simulink model "Sim_PA_DDPG"  (R2025a)
settings: Solver=ode1  StartTime=0.0  StopTime=Tf  FixedStep=Ts_Sim  RelTol=1e-3
values from neighbouring files (symbols this model uses):
  control_noise = 0.05    [DDPG_simulation.mat]    (also in Test_Pos_Att_DDPG.m)
  p_IC = IC(10)    [Test_Pos_Att_DDPG.m]
  phi_IC = IC(7)    [Test_Pos_Att_DDPG.m]
  psi_IC = IC(9)    [Test_Pos_Att_DDPG.m]
  q_IC = IC(11)    [Test_Pos_Att_DDPG.m]
  r_IC = IC(12)    [Test_Pos_Att_DDPG.m]
  state_noise = 0.05    [DDPG_simulation.mat]    (also in Test_Pos_Att_DDPG.m)
  theta_IC = IC(8)    [Test_Pos_Att_DDPG.m]
  Ts_Sim = 0.01    [DDPG_simulation.mat]    (also in Test_Pos_Att_DDPG.m)
  u_IC = IC(4)    [Test_Pos_Att_DDPG.m]
  v_IC = IC(5)    [Test_Pos_Att_DDPG.m]
  w_IC = IC(6)    [Test_Pos_Att_DDPG.m]
  x_IC = IC(1)    [Test_Pos_Att_DDPG.m]
  y_IC = IC(2)    [Test_Pos_Att_DDPG.m]
  z_IC = IC(3)    [Test_Pos_Att_DDPG.m]
undefined symbols (not defined in the file or in its folder): phi_limit, pqr_Limit, psi_dsr, psi_limit, saturation_logic, theta_limit, uvw_Limit, wind_logic, xy_Limit, z_Limit
libraries: rllib x2
settings Model: Creator=nt488543  LastModifiedBy=re606359

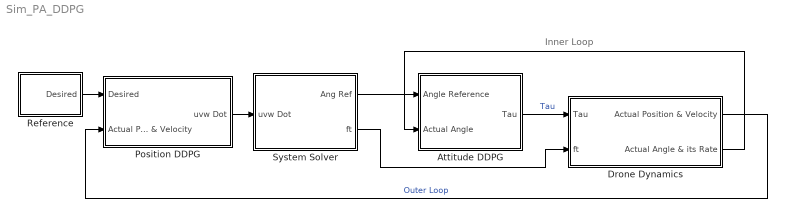
== system Sim_PA_DDPG ==
  note: Inner Loop
  Attitude DDPG : Subsystem
  Drone Dynamics : Subsystem
  Position DDPG : Subsystem
  Reference : Subsystem
  System Solver : Subsystem
  wires:
  Reference/1(Desired) -> Position DDPG/1(Desired)
  Attitude DDPG/1(Tau) -> Drone Dynamics/1(Tau)  "Tau"
  Drone Dynamics/1(Actual Position & Velocity) -> Position DDPG/2(Actual Position & Velocity)  "Outer Loop"
  Drone Dynamics/2(Actual Angle & its Rate) -> Attitude DDPG/2(Actual Angle)
  Position DDPG/1(uvw Dot) -> System Solver/1(uvw Dot)
  System Solver/1(Ang Ref) -> Attitude DDPG/1(Angle Reference)
  System Solver/2(ft) -> Drone Dynamics/2(ft)

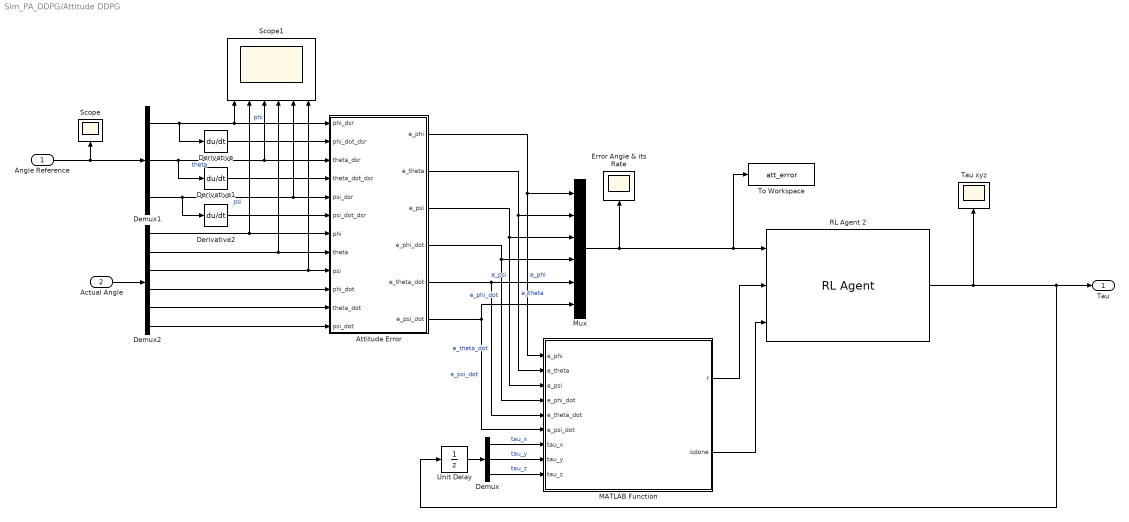
== system Sim_PA_DDPG/Attitude DDPG ==
  Angle Reference : Inport
  Actual Angle : Inport  Port=2
  Attitude Error : MATLAB Function  TreatAsAtomicUnit=on
  Demux : Demux  Outputs=3
  Demux1 : Demux  Outputs=3
  Demux2 : Demux  Outputs=6
  Derivative : Derivative
  Derivative1 : Derivative
  Derivative2 : Derivative
  Error Angle & its Rate : Scope
      settings: ActiveDisplayYMinimum=-3.5181599273654109  ActiveDisplayYMaximum=2.1435969273697308  DataLoggingVariableName=ScopeData12
  MATLAB Function : MATLAB Function  TreatAsAtomicUnit=on
  Mux : Mux  Inputs=6
  RL Agent 2 : rllib/RL Agent  Agent=agent2  ExternalActionAsInput=off  ProvideLastAction=off  ProvideCumRwd=off  TreatAsDirectFeedthrough=on  UseStrictObservationDataTypes=off
  Scope : Scope
      settings: ActiveDisplayYMinimum=-0.07573  ActiveDisplayYMaximum=0.06612  DataLoggingVariableName=ScopeData5
  Scope1 : Scope  NumInputPorts=6
      settings: ActiveDisplayYMinimum=-0.08548920227975057  ActiveDisplayYMaximum=0.079586119310867051  DataLoggingVariableName=ScopeData6
  Tau xyz : Scope
      settings: ActiveDisplayYMinimum=-2.4987406879663467  ActiveDisplayYMaximum=2.4991613775491714  DataLoggingVariableName=ScopeData11
  To Workspace : ToWorkspace  VariableName=att_error  SampleTime=Ts_Sim
  Unit Delay : UnitDelay  SampleTime=Ts_Sim  HasFrameUpgradeWarning=on
  Tau : Outport
  wires:
  MATLAB Function/1(r) -> RL Agent 2/2
  Mux/1 -> To Workspace/1, RL Agent 2/1, Error Angle & its Rate/1
  Attitude Error/1(e_phi) -> Mux/1, MATLAB Function/1(e_phi)  "e_phi"
  Attitude Error/2(e_theta) -> Mux/2, MATLAB Function/2(e_theta)  "e_theta"
  Attitude Error/3(e_psi) -> Mux/3, MATLAB Function/3(e_psi)  "e_psi"
  Attitude Error/4(e_phi_dot) -> Mux/4, MATLAB Function/4(e_phi_dot)  "e_phi_dot"
  Attitude Error/5(e_theta_dot) -> MATLAB Function/5(e_theta_dot), Mux/5  "e_theta_dot"
  Attitude Error/6(e_psi_dot) -> MATLAB Function/6(e_psi_dot), Mux/6  "e_psi_dot"
  MATLAB Function/2(isdone) -> RL Agent 2/3
  Demux/1 -> MATLAB Function/7(tau_x)  "tau_x"
  Demux/2 -> MATLAB Function/8(tau_y)  "tau_y"
  Demux/3 -> MATLAB Function/9(tau_z)  "tau_z"
  RL Agent 2/1 -> Unit Delay/1, Tau/1, Tau xyz/1
  Demux2/1 -> Scope1/2, Attitude Error/7(phi)
  Demux2/2 -> Scope1/4, Attitude Error/8(theta)
  Demux2/3 -> Attitude Error/9(psi), Scope1/6
  Demux2/4 -> Attitude Error/10(phi_dot)
  Demux2/5 -> Attitude Error/11(theta_dot)
  Demux2/6 -> Attitude Error/12(psi_dot)
  Actual Angle/1 -> Demux2/1
  Unit Delay/1 -> Demux/1
  Demux1/1 -> Derivative/1, Attitude Error/1(phi_dsr), Scope1/1  "phi"
  Demux1/3 -> Derivative2/1, Attitude Error/5(psi_dsr), Scope1/5  "psi"
  Demux1/2 -> Derivative1/1, Attitude Error/3(theta_dsr), Scope1/3  "theta"
  Angle Reference/1 -> Demux1/1, Scope/1
  Derivative/1 -> Attitude Error/2(phi_dot_dsr)
  Derivative1/1 -> Attitude Error/4(theta_dot_dsr)
  Derivative2/1 -> Attitude Error/6(psi_dot_dsr)

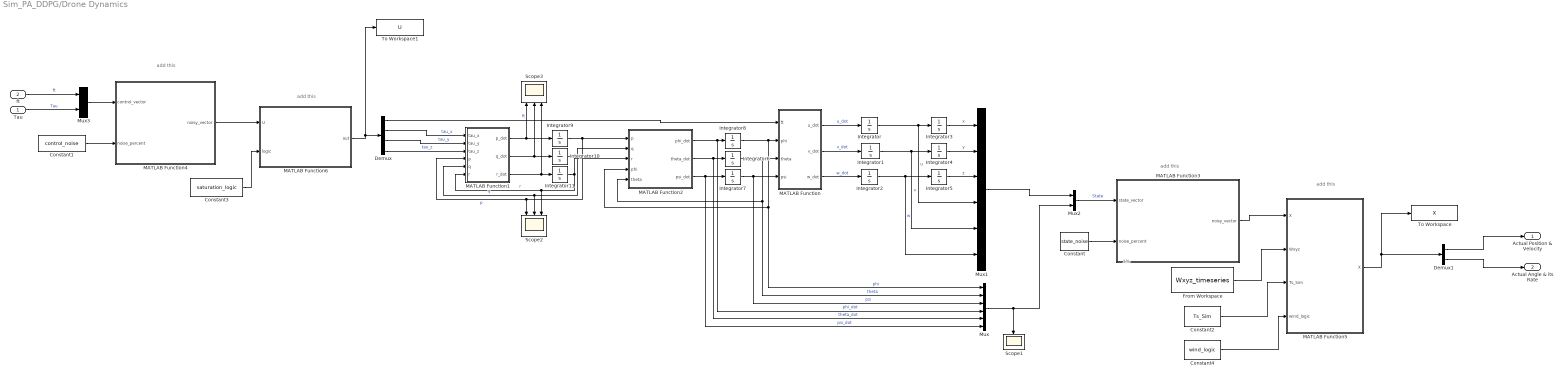
== system Sim_PA_DDPG/Drone Dynamics ==
  note: add this
  note: 1%
  note: add this
  note: add this
  note: add this
  Tau : Inport
  ft : Inport  Port=2
  Constant : Constant  Value=state_noise  SampleTime=Ts_Sim
  Constant1 : Constant  Value=control_noise
  Constant2 : Constant  Value=Ts_Sim
  Constant3 : Constant  Value=saturation_logic  SampleTime=Ts_Sim
  Constant4 : Constant  Value=wind_logic
  Demux : Demux
  Demux1 : Demux  Outputs=2
  From Workspace : FromWorkspace  VariableName=Wxyz_timeseries  SampleTime=Ts_Sim
  Integrator : Integrator  InitialCondition=u_IC  UpperSaturationLimit=uvw_Limit  LowerSaturationLimit=-uvw_Limit
  Integrator1 : Integrator  InitialCondition=v_IC  UpperSaturationLimit=uvw_Limit  LowerSaturationLimit=-uvw_Limit
  Integrator10 : Integrator  InitialCondition=q_IC  UpperSaturationLimit=pqr_Limit  LowerSaturationLimit=-pqr_Limit
  Integrator11 : Integrator  InitialCondition=r_IC  UpperSaturationLimit=pqr_Limit  LowerSaturationLimit=-pqr_Limit
  Integrator2 : Integrator  InitialCondition=w_IC  UpperSaturationLimit=uvw_Limit  LowerSaturationLimit=-uvw_Limit
  Integrator3 : Integrator  InitialCondition=x_IC  UpperSaturationLimit=xy_Limit  LowerSaturationLimit=-xy_Limit
  Integrator4 : Integrator  InitialCondition=y_IC  UpperSaturationLimit=xy_Limit  LowerSaturationLimit=-xy_Limit
  Integrator5 : Integrator  InitialCondition=z_IC  UpperSaturationLimit=z_Limit  LowerSaturationLimit=-z_Limit
  Integrator6 : Integrator  InitialCondition=theta_IC  UpperSaturationLimit=theta_limit  LowerSaturationLimit=-theta_limit  WrappedStateUpperValue=pi/2  WrappedStateLowerValue=-pi/2
  Integrator7 : Integrator  InitialCondition=psi_IC  UpperSaturationLimit=psi_limit  LowerSaturationLimit=-psi_limit
  Integrator8 : Integrator  InitialCondition=phi_IC  UpperSaturationLimit=phi_limit  LowerSaturationLimit=-phi_limit
  Integrator9 : Integrator  InitialCondition=p_IC  UpperSaturationLimit=pqr_Limit  LowerSaturationLimit=-pqr_Limit
  MATLAB Function : MATLAB Function  TreatAsAtomicUnit=on
  MATLAB Function1 : MATLAB Function  TreatAsAtomicUnit=on
  MATLAB Function2 : MATLAB Function  TreatAsAtomicUnit=on
  MATLAB Function3 : MATLAB Function  TreatAsAtomicUnit=on
  MATLAB Function4 : MATLAB Function  TreatAsAtomicUnit=on
  MATLAB Function5 : MATLAB Function  TreatAsAtomicUnit=on
  MATLAB Function6 : MATLAB Function  TreatAsAtomicUnit=on
  Mux : Mux  Inputs=6
  Mux1 : Mux  Inputs=6
  Mux2 : Mux  Inputs=2
  Mux3 : Mux  Inputs=2
  Scope1 : Scope
      settings: ActiveDisplayYMinimum=-0.79782557910284335  ActiveDisplayYMaximum=0.70695961840012789  DataLoggingVariableName=ScopeData2
  Scope2 : Scope  NumInputPorts=3
      settings: ActiveDisplayYMinimum=-0.95183  ActiveDisplayYMaximum=0.89979  DataLoggingVariableName=ScopeData3
  Scope3 : Scope  NumInputPorts=3
      settings: ActiveDisplayYMinimum=-1  ActiveDisplayYMaximum=1  DataLoggingVariableName=ScopeData4
  To Workspace : ToWorkspace  VariableName=X  SampleTime=Ts_Sim
  To Workspace1 : ToWorkspace  VariableName=U  SampleTime=Ts_Sim
  Actual Position & Velocity : Outport
  Actual Angle & its Rate : Outport  Port=2
  wires:
  Integrator4/1 -> Mux1/2  "y"
  MATLAB Function1/3(r_dot) -> Scope3/3, Integrator11/1
  MATLAB Function1/1(p_dot) -> Scope3/1, Integrator9/1
  Integrator3/1 -> Mux1/1  "x"
  Integrator5/1 -> Mux1/3  "z"
  Integrator1/1 -> Mux1/5, Integrator4/1  "v"
  ft/1 -> Mux3/1  "ft"
  Demux/3 -> MATLAB Function1/2(tau_y)  "tau_y"
  Integrator9/1 -> MATLAB Function1/4(p), Scope2/1, MATLAB Function2/1(p)  "p"
  Integrator11/1 -> MATLAB Function1/6(r), Scope2/3, MATLAB Function2/3(r)  "r"
  Integrator2/1 -> Mux1/6, Integrator5/1  "w"
  Integrator/1 -> Mux1/4, Integrator3/1  "u"
  Tau/1 -> Mux3/2  "Tau"
  Integrator7/1 -> Mux/3, MATLAB Function/4(psi)  "psi"
  Integrator8/1 -> Mux/1, MATLAB Function2/4(phi), MATLAB Function/2(phi)  "phi"
  Integrator6/1 -> MATLAB Function/3(theta), Mux/2, MATLAB Function2/5(theta)  "theta"
  Integrator10/1 -> MATLAB Function2/2(q), MATLAB Function1/5(q), Scope2/2  "q"
  Demux/4 -> MATLAB Function1/3(tau_z)  "tau_z"
  Mux/1 -> Scope1/1, Mux2/2
  MATLAB Function/3(w_dot) -> Integrator2/1  "w_dot"
  MATLAB Function/1(u_dot) -> Integrator/1  "u_dot"
  MATLAB Function/2(v_dot) -> Integrator1/1  "v_dot"
  MATLAB Function1/2(q_dot) -> Scope3/2, Integrator10/1
  Demux/2 -> MATLAB Function1/1(tau_x)  "tau_x"
  MATLAB Function2/1(phi_dot) -> Mux/4, Integrator8/1  "phi_dot"
  MATLAB Function2/2(theta_dot) -> Mux/5, Integrator6/1  "theta_dot"
  MATLAB Function2/3(psi_dot) -> Mux/6, Integrator7/1  "psi_dot"
  Mux2/1 -> MATLAB Function3/1(state_vector)  "State"
  MATLAB Function3/1(noisy_vector) -> MATLAB Function5/1("X ")
  Mux1/1 -> Mux2/1
  Constant/1 -> MATLAB Function3/2(noise_percent)
  Mux3/1 -> MATLAB Function4/1(control_vector)
  Constant1/1 -> MATLAB Function4/2(noise_percent)
  MATLAB Function4/1(noisy_vector) -> MATLAB Function6/1(U)
  Demux/1 -> MATLAB Function/1(ft)  "ft"
  From Workspace/1 -> MATLAB Function5/2(Wxyz)
  Demux1/2 -> Actual Angle & its Rate/1
  Demux1/1 -> Actual Position & Velocity/1
  Constant2/1 -> MATLAB Function5/3(Ts_Sim)
  MATLAB Function5/1(X) -> To Workspace/1, Demux1/1
  MATLAB Function6/1(out) -> To Workspace1/1, Demux/1
  Constant3/1 -> MATLAB Function6/2(logic)
  Constant4/1 -> MATLAB Function5/4(wind_logic)

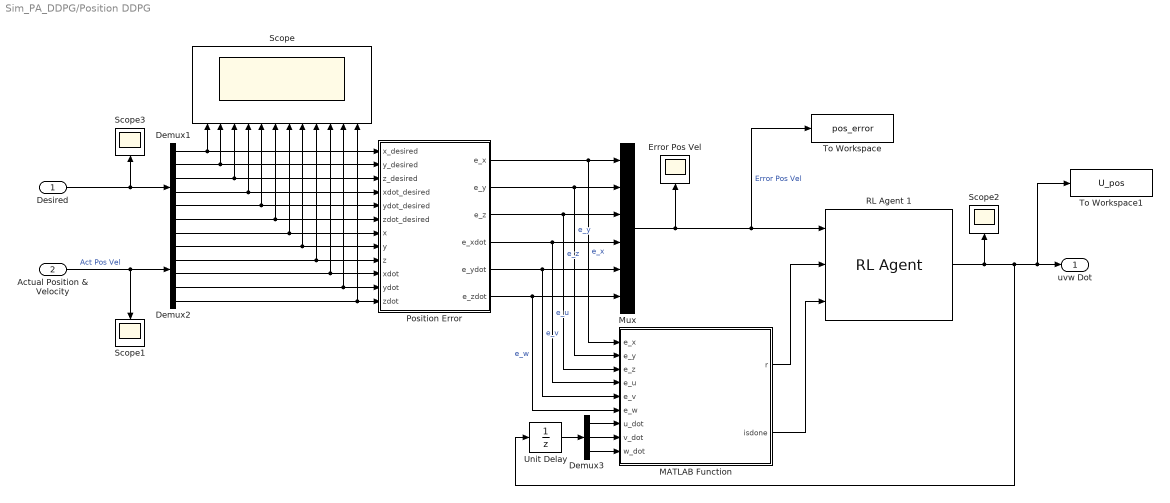
== system Sim_PA_DDPG/Position DDPG ==
  Desired : Inport
  Actual Position & Velocity : Inport  Port=2
  Demux1 : Demux  Outputs=6
  Demux2 : Demux  Outputs=6
  Demux3 : Demux  Outputs=3
  Error Pos Vel : Scope
      settings: ActiveDisplayYMinimum=-1.3710264936743408  ActiveDisplayYMaximum=0.56946492466600562  DataLoggingVariableName=Error
  MATLAB Function : MATLAB Function  TreatAsAtomicUnit=on
  Mux : Mux  Inputs=6
  Position Error : MATLAB Function  TreatAsAtomicUnit=on
  RL Agent 1 : rllib/RL Agent  Agent=agent  ExternalActionAsInput=off  ProvideLastAction=off  ProvideCumRwd=off  TreatAsDirectFeedthrough=on  UseStrictObservationDataTypes=off
  Scope : Scope  NumInputPorts=12
      settings: ActiveDisplayYMinimum=-64.8105630976365  ActiveDisplayYMaximum=12.296113517917625  DataLoggingVariableName=Difference
  Scope1 : Scope
      settings: ActiveDisplayYMinimum=-34.05865723917438  ActiveDisplayYMaximum=6.4948745222233439  DataLoggingVariableName=Actual
  Scope2 : Scope
      settings: ActiveDisplayYMinimum=-2.3417  ActiveDisplayYMaximum=1.0752  DataLoggingVariableName=ScopeData4
  Scope3 : Scope
      settings: ActiveDisplayYMinimum=-34.036737735877395  ActiveDisplayYMaximum=6.4906396228965306  DataLoggingVariableName=Ref
  To Workspace : ToWorkspace  VariableName=pos_error  SampleTime=Ts_Sim
  To Workspace1 : ToWorkspace  VariableName=U_pos  SampleTime=Ts_Sim
  Unit Delay : UnitDelay  SampleTime=Ts_Sim  HasFrameUpgradeWarning=on
  uvw Dot : Outport
  wires:
  MATLAB Function/1(r) -> RL Agent 1/2
  Mux/1 -> To Workspace/1, RL Agent 1/1, Error Pos Vel/1  "Error Pos Vel"
  RL Agent 1/1 -> To Workspace1/1, uvw Dot/1, Unit Delay/1, Scope2/1
  Position Error/1(e_x) -> MATLAB Function/1(e_x), Mux/1  "e_x"
  Position Error/2(e_y) -> MATLAB Function/2(e_y), Mux/2  "e_y"
  Position Error/3(e_z) -> Mux/3, MATLAB Function/3(e_z)  "e_z"
  Position Error/4(e_xdot) -> MATLAB Function/4(e_u), Mux/4  "e_u"
  Position Error/5(e_ydot) -> MATLAB Function/5(e_v), Mux/5  "e_v"
  Position Error/6(e_zdot) -> MATLAB Function/6(e_w), Mux/6  "e_w"
  MATLAB Function/2(isdone) -> RL Agent 1/3
  Demux1/1 -> Position Error/1(x_desired), Scope/1
  Demux1/2 -> Position Error/2(y_desired), Scope/2
  Demux1/3 -> Position Error/3(z_desired), Scope/3
  Demux1/4 -> Position Error/4(xdot_desired), Scope/4
  Demux1/5 -> Position Error/5(ydot_desired), Scope/5
  Demux1/6 -> Position Error/6(zdot_desired), Scope/6
  Desired/1 -> Scope3/1, Demux1/1
  Demux2/1 -> Position Error/7(x), Scope/7
  Demux2/2 -> Position Error/8(y), Scope/8
  Demux2/3 -> Position Error/9(z), Scope/9
  Demux2/4 -> Position Error/10(xdot), Scope/10
  Demux2/5 -> Position Error/11(ydot), Scope/11
  Demux2/6 -> Scope/12, Position Error/12(zdot)
  Actual Position & Velocity/1 -> Demux2/1, Scope1/1  "Act Pos Vel"
  Demux3/1 -> MATLAB Function/7(u_dot)
  Demux3/2 -> MATLAB Function/8(v_dot)
  Demux3/3 -> MATLAB Function/9(w_dot)
  Unit Delay/1 -> Demux3/1

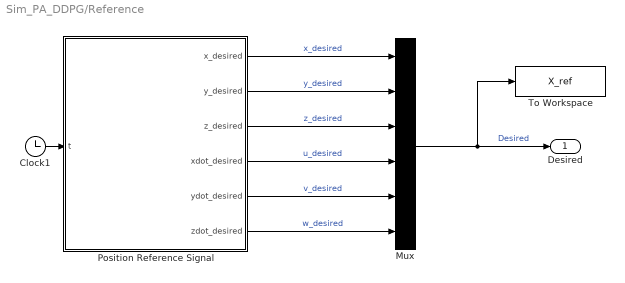
== system Sim_PA_DDPG/Reference ==
  Clock1 : Clock
  Mux : Mux  Inputs=6
  Position Reference Signal : MATLAB Function  TreatAsAtomicUnit=on
  To Workspace : ToWorkspace  VariableName=X_ref  SampleTime=Ts_Sim
  Desired : Outport
  wires:
  Position Reference Signal/2(y_desired) -> Mux/2  "y_desired"
  Position Reference Signal/4(xdot_desired) -> Mux/4  "u_desired"
  Position Reference Signal/6(zdot_desired) -> Mux/6  "w_desired"
  Clock1/1 -> Position Reference Signal/1(t)
  Position Reference Signal/3(z_desired) -> Mux/3  "z_desired"
  Position Reference Signal/1(x_desired) -> Mux/1  "x_desired"
  Position Reference Signal/5(ydot_desired) -> Mux/5  "v_desired"
  Mux/1 -> To Workspace/1, Desired/1  "Desired"

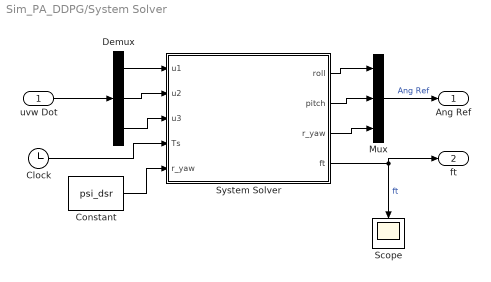
== system Sim_PA_DDPG/System Solver ==
  uvw Dot : Inport
  Clock : Clock
  Constant : Constant  Value=psi_dsr
  Demux : Demux  Outputs=3
  Mux : Mux  Inputs=3
  Scope : Scope
      settings: ActiveDisplayYMinimum=5.5477079741609581  ActiveDisplayYMaximum=13.965080226414941
  System Solver : MATLAB Function  TreatAsAtomicUnit=on
  Ang Ref : Outport
  ft : Outport  Port=2
  wires:
  System Solver/2(pitch) -> Mux/2
  Demux/1 -> System Solver/1(u1)
  System Solver/3(r_yaw) -> Mux/3
  Demux/2 -> System Solver/2(u2)
  System Solver/1(roll) -> Mux/1
  Demux/3 -> System Solver/3(u3)
  System Solver/4(ft) -> ft/1, Scope/1  "ft"
  Clock/1 -> System Solver/4(Ts)
  Mux/1 -> Ang Ref/1  "Ang Ref"
  uvw Dot/1 -> Demux/1
  Constant/1 -> System Solver/5("r_yaw ")

== matlab function Sim_PA_DDPG/Reference/Position Reference Signal ==
  data: t input; x_desired output; y_desired output; z_desired output; xdot_desired output; ydot_desired output; zdot_desired output
function [x_desired, y_desired, z_desired, xdot_desired, ydot_desired, zdot_desired] = trajectory_generator(t)

    x_desired    = 9.81 * (1-exp(-0.01*t)) * cos(0.2*t);
    xdot_desired = 9.81 * ( (0.01*exp(-0.01*t)*cos(0.2*t)) - (0.2*(1-exp(-0.01*t))*sin(0.2*t)) );

    y_desired    = 9.81 * (1-exp(-0.01*t)) * sin(0.2*t);
    ydot_desired = 9.81 * ( (0.01*exp(-0.01*t)*sin(0.2*t)) + (0.2*(1-exp(-0.01*t))*cos(0.2*t)) );

    z_desired    = -1*t;
    zdot_desired = -1;

end


% ref = @(t) [(1-exp(-0.01*t))*9.81*cos(0.2*t);
%             (1-exp(-0.01*t))*9.81*sin(0.2*t);
%             -.1*t];


 % x_desired    = 9.81 * (1-exp(-0.01*t)) * cos(0.2*t);
 %    xdot_desired = 9.81 * ( (0.01*exp(-0.01*t)*cos(0.2*t)) - (0.2*(1-exp(-0.01*t))*sin(0.2*t)) );
 % 
 %    y_desired    = 9.81 * (1-exp(-0.01*t)) * sin(0.2*t);
 %    ydot_desired = 9.81 * ( (0.01*exp(-0.01*t)*sin(0.2*t)) + (0.2*(1-exp(-0.01*t))*cos(0.2*t)) );
 % 
 %    z_desired    = -0.1*t;
 %    zdot_desired = -0.1;

== matlab function Sim_PA_DDPG/System Solver/System Solver ==
  data: roll output; pitch output; r_yaw output; ft output; u1 input; u2 input; u3 input; Ts input; r_yaw input
function [roll, pitch, r_yaw, ft ] = system_solver(u1, u2, u3, Ts, r_yaw)

    m = 1; g = 9.81;
    
    ft = m * sqrt( u1^2 + u2^2 + (u3-g)^2 );

    % a = sin(r_yaw);
    % b = cos(r_yaw);
    % 
    % A = u1 / (u3);
    % B = u2 / (u3);
    % C = (a*A - b*B) / ( (a^2) + (b^2)) ;
    % 
    % roll = atan( (B + b*C) / a );
    % pitch = atan( C * cos(roll) );

    roll = asin( (u2*m) / ft );
    pitch = asin( (-u1*m) / (ft*cos(roll)) );
    r_yaw = 0;

    % Smoothing Factor ( Use exponential decay, just to start from zero )
    % roll = roll * (1-exp(-Ts));
    % pitch = pitch * (1-exp(-Ts));
    % r_yaw = r_yaw * (1-exp(-Ts));

    % Saturation
    if roll > pi/10
        roll = pi/10;
    elseif roll < -pi/10
        roll = -pi/10;
    end

    if pitch > pi/10
        pitch = pi/10;
    elseif pitch < -pi/10
        pitch = -pi/10;
    end

end

% function [ft, pitch, roll] = system_solve(u1, u2, u3, psi, m) % u1 = ux , u2 = uy , u3 = uz - g  
%     if psi <= 0.001 && psi >= -0.001
%         psi = 0.001;
%     end
%     a = sin(psi);
%     b = cos(psi);
% 
%     A = u1 / (u3);
%     B = u2 / (u3);
%     C = (a*A - b*B) / ( (a^2) + (b^2)) ;
% 
%     roll = atan( (B + b*C) / a );
%     pitch = atan( C * cos(roll) );
% 
%     % saftey limit threshold on desired pitch and roll
%     if pitch>pi/4
%         pitch = pi/4;
%     elseif pitch<-pi/4
%         pitch = -pi/4;
%     end
%     if roll>pi/4
%         roll = pi/4;
%     elseif roll<-pi/4
%         roll = -pi/4;
%     end
%     ft = ( m / (cos(pitch)*cos(roll)) ) * (-u3); 
% end

== matlab function Sim_PA_DDPG/Attitude DDPG/Attitude Error ==
  data: phi_dsr input; phi_dot_dsr input; theta_dsr input; theta_dot_dsr input; psi_dsr input; psi_dot_dsr input; phi input; theta input; psi input; e_phi output; e_theta output; e_psi output; phi_dot input; theta_dot input; psi_dot input; e_phi_dot output; e_theta_dot output; e_psi_dot output
function [ e_phi, e_theta, e_psi, e_phi_dot, e_theta_dot, e_psi_dot ] = calculate_errors(phi_dsr, phi_dot_dsr, theta_dsr, theta_dot_dsr, psi_dsr, psi_dot_dsr, phi, theta, psi, phi_dot, theta_dot, psi_dot)
   
    e_phi = phi_dsr - phi;
    e_theta = theta_dsr - theta;
    e_psi = psi_dsr - psi;

    e_phi_dot = phi_dot_dsr - phi_dot;
    e_theta_dot = theta_dot_dsr - theta_dot;
    e_psi_dot = psi_dot_dsr - psi_dot;

end

== matlab function Sim_PA_DDPG/Position DDPG/Position Error ==
  data: x_desired input; y_desired input; z_desired input; xdot_desired input; ydot_desired input; zdot_desired input; x input; y input; z input; e_x output; e_y output; e_z output; xdot input; ydot input; zdot input; e_xdot output; e_ydot output; e_zdot output
function [e_x, e_y, e_z, e_xdot, e_ydot, e_zdot] = ...
      calculate_errors(x_desired, y_desired, z_desired, ...
      xdot_desired, ydot_desired, zdot_desired, ...
      x,y,z, xdot,ydot,zdot)

    e_x    = x_desired - x;
    e_y    = y_desired - y;
    e_z    = z_desired - z;
    e_xdot = xdot_desired - xdot;
    e_ydot = ydot_desired - ydot;
    e_zdot = zdot_desired - zdot;
    
end

% formal is Actual - Reference

== matlab function Sim_PA_DDPG/Position DDPG/MATLAB Function ==
  data: e_x input; r output; e_y input; e_z input; e_u input; e_v input; e_w input; u_dot input; v_dot input; w_dot input; isdone output
function [r,isdone] = calculate_reward(e_x, e_y, e_z, e_u, e_v, e_w, u_dot, v_dot, w_dot)

    r = -    1*( abs(e_x)   + abs(e_y)   + abs(e_z) ) ...
        -  0.1*( abs(e_u)   + abs(e_v)   + abs(e_w) ) ...
        - 0.01*( abs(u_dot) + abs(v_dot) + abs(w_dot) );
    
   isdone = 0;
   
end

== matlab function Sim_PA_DDPG/Attitude DDPG/MATLAB Function ==
  data: e_phi input; r output; e_theta input; e_psi input; e_phi_dot input; e_theta_dot input; e_psi_dot input; tau_x input; tau_y input; tau_z input; isdone output
function [r,isdone] = calculate_reward(e_phi, e_theta, e_psi, e_phi_dot, e_theta_dot, e_psi_dot, tau_x, tau_y, tau_z )

    Error_Angle      =    2*( abs(e_phi)     +  abs(e_theta)     + abs(e_psi) );
    Error_Angle_Rate =  0.1*( abs(e_phi_dot) +  abs(e_theta_dot) + abs(e_psi_dot) );
    Action           = 0.01*( abs(tau_x)     +  abs(tau_y)       + abs(tau_z) );

    r = - Error_Angle - Error_Angle_Rate - Action;

    isdone = (abs(e_phi) > 100) || (abs(e_theta) > 100) || (abs(e_psi) > 100);
end

== matlab function Sim_PA_DDPG/Drone Dynamics/MATLAB Function1 ==
  data: tau_x input; p_dot output; tau_y input; tau_z input; p input; q_dot output; r_dot output; q input; r input
function [p_dot, q_dot, r_dot] = fcn(tau_x,tau_y,tau_z,p,q,r)

Ix = 0.3; Iy = 0.4; Iz = 0.5; 

p_dot = ((Iy-Iz)*q*r/Ix)  + tau_x/Ix;
q_dot = ((Iz-Ix)*p*r/Iy)  + tau_y/Iy;
r_dot = ((Ix-Iy)*p*q/Iz)  + tau_z/Iz;


end

== matlab function Sim_PA_DDPG/Drone Dynamics/MATLAB Function ==
  data: ft input; u_dot output; phi input; theta input; psi input; v_dot output; w_dot output
function [u_dot, v_dot, w_dot] = fcn(ft,phi,theta,psi)

m = 1; g = 9.81;

u_dot = -(ft/m)*( sin(phi)*sin(psi) + cos(phi)*cos(psi)*sin(theta) ); 
v_dot = -(ft/m)*( cos(phi)*sin(psi)*sin(theta) - cos(psi)*sin(phi));
w_dot = g-(ft/m)*( cos(phi)*cos(theta) );

end

== matlab function Sim_PA_DDPG/Drone Dynamics/MATLAB Function2 ==
  data: p input; q input; r input; phi_dot output; phi input; theta input; theta_dot output; psi_dot output
function [phi_dot, theta_dot, psi_dot] = fcn(p,q,r, phi,theta)

    phi_dot   = p + (q*sin(phi)*tan(theta)) + (r*cos(phi)*tan(theta));
    theta_dot = (q*cos(phi)) - (r*sin(phi));
    psi_dot   = (q*sin(phi)/cos(theta)) + (r*cos(phi)/cos(theta));

end



    % if theta == deg2rad(90) || theta == deg2rad(-90)
    %    theta = sign(theta)*deg2rad(89.9); 
    % end

% 89.9 value is fixed. 
% if change to 89.99, phi_dot and psi_dot value will explode.

== matlab function Sim_PA_DDPG/Drone Dynamics/MATLAB Function3 ==
  settings: updateMethod=DISCRETE
  data: state_vector input; noisy_vector output; noise_percent input
function noisy_vector = add_state_noise(state_vector,noise_percent)

    sensor_uncert = [0.02, 0.02, 0.05, 0.05, 0.05, 0.05, 0.15, 0.15, 0.5, 0.005, 0.005, 0.005]';
  
    noise = (noise_percent) * sensor_uncert .* randn(size(state_vector)); % 0.01 usually add noise_percent 1 2 3 4 5
    noisy_vector = state_vector + noise;

end

== matlab function Sim_PA_DDPG/Drone Dynamics/MATLAB Function4 ==
  settings: updateMethod=DISCRETE
  data: control_vector input; noisy_vector output; noise_percent input
function noisy_vector = add_control_noise(control_vector, noise_percent)

    L = 0.2;
    % drag = 0.02; % (drag coef)
    max_Ft = 2*9.81;
    Tmax = max_Ft/4;
    Max_torque = Tmax*L*2;
    actuator_uncert = [0.1*max_Ft, 0.01*Max_torque, 0.01*Max_torque, 0.02*Max_torque]';
    
    noise = (noise_percent) * actuator_uncert .* randn(size(control_vector)); % noise_percent 1 2 3 4 5
    noisy_vector = control_vector + noise;
    
end

== matlab function Sim_PA_DDPG/Drone Dynamics/MATLAB Function5 ==
  data: X input; Wxyz input; X output; Ts_Sim input; wind_logic input
function X = wind_f_m( X,Wxyz, Ts_Sim,  wind_logic)

    Cd = [.8; 0.8;1.2]; % Drag coefficient
    L = 0.2; % Half arm length (m)
    h = 0.05;
    A = [L*2*h, L*2*h, 2*L*L]; % Approximate frontal areas [x, y, z] in m^2
    r = [ L,  L, -L, -L;   % X positions of motors
          L, -L, -L,  L;   % Y positions of motors
          0,  0,  0,  0 ]; % Z positions (motors at same height)
    rho = 1.225; % Air density (kg/m^3)

    Ix = 0.3; Iy = 0.4; Iz = 0.5; m = 1;
    if wind_logic ==1
        R = eul2rotm_zyx( X(7), X(8), X(9) );
        Wxyz_body = R'*Wxyz;
        V_rel = X(4:6) - Wxyz_body;
        F_wind = -0.5 * rho * Cd .*diag(A) * (V_rel .* abs(V_rel)); % Compute wind forces
        
        F_wind_motors = repmat(F_wind, 1, 4) + 0.01*randn(3,4);
    
        M_wind_motors = cross(r, F_wind_motors, 1);
        M_wind = sum(M_wind_motors, 2);  
        
        accn_dist = F_wind/m;
        alpha_dist=    [M_wind(1)/Ix;
                        M_wind(2)/Iy;
                        M_wind(3)/Iz];
    
        X = X + Ts_Sim * [0;0;0;
                         accn_dist;
                         0;0;0;
                         alpha_dist];
    end
end

== matlab function Sim_PA_DDPG/Drone Dynamics/MATLAB Function6 ==
  data: U input; out output; logic input
% saturation function
function out = saturate_controls(U, logic)

    if logic == 1

        ft = U(1);
        torques = [U(2); U(3); U(4)];
        m = 1;
        g = 9.81;
        L = 0.2;
        drag = 0.02; % (drag coef)
        max_Ft = 2*m*g;
        Tmin = 0;
        Tmax = max_Ft/4;
        max_torque = Tmax*L*2;
        max_yaw_torque = 0.7*max_torque;

        % saturate the torques to the max torque the drone can produce
        for p = 1:2 % sat the first 2
            if torques(p) > max_torque
                torques(p) = max_torque;
            elseif torques(p) < -max_torque
                torques(p) = -max_torque;
            end
        end
        if torques(3) > max_yaw_torque
            torques(3) = max_yaw_torque;
        elseif torques(3) < -max_yaw_torque
            torques(3) = -max_yaw_torque;
        end
        % solve for the thrust of each motor given those torques
        T1 = (ft - torques(1)/(2*L) - torques(2)/(2*L) + torques(3)/(4*drag)) / 4;
        T2 = (ft - torques(1)/(2*L) + torques(2)/(2*L) + torques(3)/(4*drag)) / 4;
        T3 = (ft + torques(1)/(2*L) - torques(2)/(2*L) - torques(3)/(4*drag)) / 4;
        T4 = (ft + torques(1)/(2*L) + torques(2)/(2*L) - torques(3)/(4*drag)) / 4;
        each_motor_thrust = [T1;T2;T3;T4];

        % saturate each motor thrust to its bounded values
        for j = 1:4
            if each_motor_thrust(j) > Tmax
                each_motor_thrust(j) = Tmax;
            elseif each_motor_thrust(j) < Tmin
                each_motor_thrust(j) = Tmin;
            end
        end

        ft = sum(each_motor_thrust);

        if ft>max_Ft
            ft = max_Ft;
        elseif ft<0
            ft = 0;
        end

        out = [ft; torques];

    else
    
        out = U;
    
    end


end
